simulink model "Sim_Ex11"  (R2017a)
settings: Solver=VariableStepAuto  StartTime=0.0  StopTime=10.0  RelTol=1e-3
values from neighbouring files (symbols this model uses):
  L = 1    [A_Ex11.m]
  R = 1    [A_Ex11.m]
settings Model: Creator=KYC  LastModifiedBy=KYC

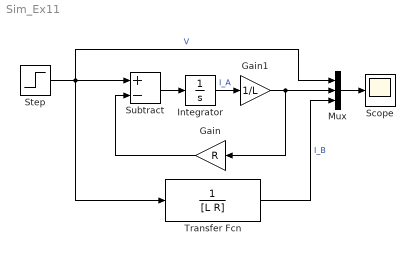
== system Sim_Ex11 ==
  Gain : Gain  Gain=R
  Gain1 : Gain  Gain=1/L
  Integrator : Integrator
  Mux : Mux  Inputs=3
  Scope : Scope
  Step : Step  SampleTime=0
  Subtract : Sum  Inputs=+-
  Transfer Fcn : TransferFcn  Denominator=[L R]
  wires:
  Gain/1 -> Subtract/2
  Step/1 -> Mux/1, Transfer Fcn/1, Subtract/1  "V"
  Integrator/1 -> Gain1/1  "I_A"
  Subtract/1 -> Integrator/1
  Mux/1 -> Scope/1
  Transfer Fcn/1 -> Mux/3  "I_B"
  Gain1/1 -> Gain/1, Mux/2
